simulink model "PSB_FPGAdesign8_model"  (R2021a)
settings: Solver=VariableStepAuto  StartTime=0.0  StopTime=3000  RelTol=1e-3
values from neighbouring files (symbols this model uses):
  n_channel = 1024    [PSB3_0_script.m]    (also in PSB_FPGAdesign8_script.m)
  parallel_factor = 4    [PSB3_0_script.m]    (also in PSB_FPGAdesign8_script.m)
libraries: xbsIndex_r4 x1089, xrbsSSR_Library x150, dspsrcs4 x48
(part 6 of 7)

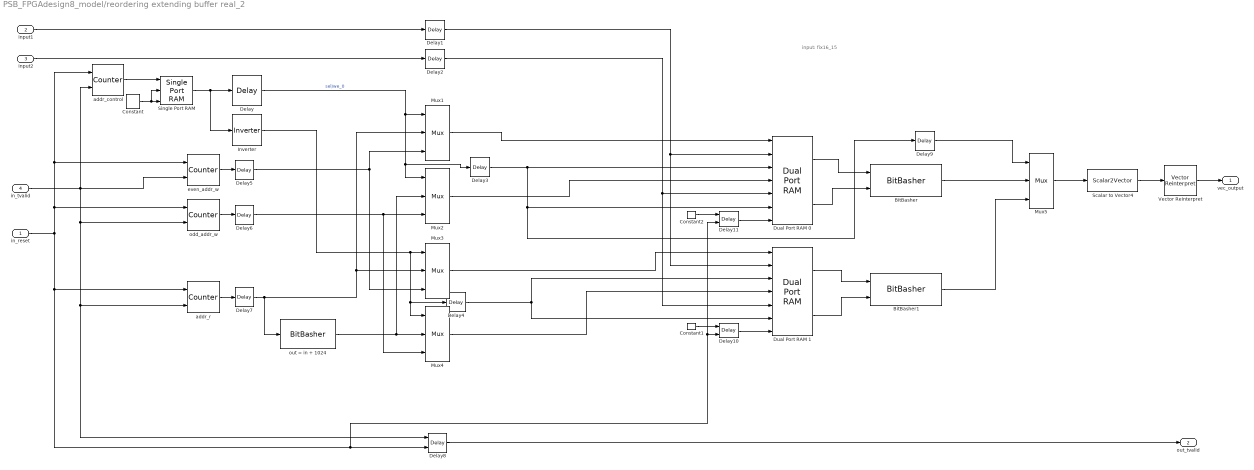
== system PSB_FPGAdesign8_model/reordering extending buffer real_2 ==
  note: input: fix16_15
  in_reset : Inport
  input1 : Inport  Port=2
  input2 : Inport  Port=3
  in_tvalid : Inport  Port=4
  BitBasher : xbsIndex_r4/BitBasher  bitexpr=out = {8{b,a}}  display_expr=on  sr_1=out  arith_type1=Unsigned  bin_pt1=0  sr_2=2  arith_type2=Unsigned  bin_pt2=0  sr_3=3  arith_type3=Unsigned  bin_pt3=0  sr_4=4  arith_type4=Unsigned  bin_pt4=0  dbl_ovrd=off  block_type=bitbasher
  BitBasher1 : xbsIndex_r4/BitBasher  bitexpr=out = {8{b,a}}  display_expr=on  sr_1=out  arith_type1=Unsigned  bin_pt1=0  sr_2=2  arith_type2=Unsigned  bin_pt2=0  sr_3=3  arith_type3=Unsigned  bin_pt3=0  sr_4=4  arith_type4=Unsigned  bin_pt4=0  dbl_ovrd=off  block_type=bitbasher
  Constant : xbsIndex_r4/Constant  const=0  gui_display_data_type=Boolean  arith_type=Boolean  n_bits=16  bin_pt=14  preci_type=Single  exp_width=8  frac_width=24  explicit_period=on  period=1  equ=P=C  opselect=C  inp2=PCIN>>17  opr=+  inp1=P  carry=CIN  dbl_ovrd=off  block_type=constant
  Constant1 : xbsIndex_r4/Constant  const=1  gui_display_data_type=Boolean  arith_type=Boolean  n_bits=16  bin_pt=14  preci_type=Single  exp_width=8  frac_width=24  explicit_period=on  period=1  equ=P=C  opselect=C  inp2=PCIN>>17  opr=+  inp1=P  carry=CIN  dbl_ovrd=off  block_type=constant
  Constant2 : xbsIndex_r4/Constant  const=1  gui_display_data_type=Boolean  arith_type=Boolean  n_bits=16  bin_pt=14  preci_type=Single  exp_width=8  frac_width=24  explicit_period=on  period=1  equ=P=C  opselect=C  inp2=PCIN>>17  opr=+  inp1=P  carry=CIN  dbl_ovrd=off  block_type=constant
  Delay{,3..4,9} (4 alike) : xbsIndex_r4/Delay  rst=off  infoeditControl=Selection of Reset will increase slice count due to use of real FFs and instead of SRLs  en=off  latency=1  reg_retiming=off  dbl_ovrd=off  block_type=delay
  Delay1 : xbsIndex_r4/Delay  rst=off  infoeditControl=Selection of Reset will increase slice count due to use of real FFs and instead of SRLs  en=off  latency=3  reg_retiming=off  dbl_ovrd=off  block_type=delay
  Delay10 : xbsIndex_r4/Delay  rst=on  infoeditControl=Selection of Reset will increase slice count due to use of real FFs and instead of SRLs  en=off  latency=1000  reg_retiming=off  dbl_ovrd=off  block_type=delay
  Delay11 : xbsIndex_r4/Delay  rst=on  infoeditControl=Selection of Reset will increase slice count due to use of real FFs and instead of SRLs  en=off  latency=1000  reg_retiming=off  dbl_ovrd=off  block_type=delay
  Delay2 : xbsIndex_r4/Delay  rst=off  infoeditControl=Selection of Reset will increase slice count due to use of real FFs and instead of SRLs  en=off  latency=3  reg_retiming=off  dbl_ovrd=off  block_type=delay
  Delay5 : xbsIndex_r4/Delay  rst=off  infoeditControl=Selection of Reset will increase slice count due to use of real FFs and instead of SRLs  en=off  latency=2  reg_retiming=off  dbl_ovrd=off  block_type=delay
  Delay6 : xbsIndex_r4/Delay  rst=off  infoeditControl=Selection of Reset will increase slice count due to use of real FFs and instead of SRLs  en=off  latency=2  reg_retiming=off  dbl_ovrd=off  block_type=delay
  Delay7 : xbsIndex_r4/Delay  rst=off  infoeditControl=Selection of Reset will increase slice count due to use of real FFs and instead of SRLs  en=off  latency=2  reg_retiming=off  dbl_ovrd=off  block_type=delay
  Delay8 : xbsIndex_r4/Delay  rst=on  infoeditControl=Selection of Reset will increase slice count due to use of real FFs and instead of SRLs  en=off  latency=4+1024/parallel_factor+1 - 2  reg_retiming=off  dbl_ovrd=off  block_type=delay
  Dual Port RAM 0 : xbsIndex_r4/Dual Port RAM  depth=2048/parallel_factor  initVector=1  distributed_mem=Block RAM  init_a=0  init_b=0  rst_a=off  rst_b=off  en_a=off  en_b=on  latency=1  write_mode_A=Read Before Write  write_mode_B=Read Before Write  optimize=Area  dbl_ovrd=off  simulation_type=fast_sim  block_type=dpram
  Dual Port RAM 1 : xbsIndex_r4/Dual Port RAM  depth=2048/parallel_factor  initVector=1  distributed_mem=Block RAM  init_a=0  init_b=0  rst_a=off  rst_b=off  en_a=off  en_b=on  latency=1  write_mode_A=Read Before Write  write_mode_B=Read Before Write  optimize=Area  dbl_ovrd=off  simulation_type=fast_sim  block_type=dpram
  Inverter : xbsIndex_r4/Inverter  en=off  latency=1  dbl_ovrd=off  block_type=inv
  Mux{1..4} (4 alike) : xbsIndex_r4/Mux  inputs=2  en=off  latency=1  precision=Full  arith_type=Unsigned  n_bits=16  bin_pt=14  quantization=Truncate  overflow=Wrap  dbl_ovrd=off  block_type=mux
  Mux5 : xbsIndex_r4/Mux  inputs=2  en=off  latency=1  precision=User Defined  arith_type=Unsigned  n_bits=256  bin_pt=0  quantization=Truncate  overflow=Flag as error  dbl_ovrd=off  block_type=mux
  Scalar to Vector4 : xrbsSSR_Library/Scalar2Vector  Width=16  sg_ssr=16  sg_ssr_prev=16  sg_ssr_name=vect_Scalar2Vector  block_type=scalar2vector_ssr
      settings: SourceProductName=Xilinx SSR Blockset
  Single Port RAM : xbsIndex_r4/Single Port RAM  depth=2048/parallel_factor  initVector=[ones(1,1024/parallel_factor), zeros(1,1024/parallel_factor)]  distributed_mem=Block RAM  write_mode=Read Before Write  rst=off  init_reg=0  en=off  optimize_latency=off  latency=1  optimize=Area  dbl_ovrd=off  simulation_type=fast_sim  block_type=spram
  Vector Reinterpret : xrbsSSR_Library/Vector Reinterpret  sg_ssr=16  sg_ssr_prev=16  force_arith_type=on  arith_type="Signed  (2's comp)"  force_bin_pt=on  bin_pt=15  block_type=reinterpret_ssr
      settings: SourceProductName=Xilinx SSR Blockset  infoedit="The Vector Reinterpret block Changes vector input signal type without altering the binary representation. You can change the signal between signed and unsigned, and relocate the binary point.<br><br>Hardware notes: In hardware this block costs nothing.<br><br>Example:  Suppose the input is 6 bits wide, signed, with 2 fractional bits, and the output is forced to unsigned with 0 fractional bits.  Then an input of -2.0 (1110.00 in binary 2's complement) becomes an output of 56 (111000 in binary)."
  addr_control : xbsIndex_r4/Counter  cnt_type=Free Running  cnt_to=Inf  operation=Up  start_count=0  cnt_by_val=1  arith_type=Unsigned  n_bits=11-2  bin_pt=0  load_pin=off  rst=on  en=on  explicit_period=on  period=1  use_behavioral_HDL=off  implementation=Fabric  dbl_ovrd=off  block_type=counter
  addr_r : xbsIndex_r4/Counter  cnt_type=Free Running  cnt_to=Inf  operation=Up  start_count=0  cnt_by_val=1  arith_type=Unsigned  n_bits=10-2  bin_pt=0  load_pin=off  rst=on  en=on  explicit_period=on  period=1  use_behavioral_HDL=off  implementation=Fabric  dbl_ovrd=off  block_type=counter
  even_addr_w : xbsIndex_r4/Counter  cnt_type=Free Running  cnt_to=Inf  operation=Up  start_count=0  cnt_by_val=2  arith_type=Unsigned  n_bits=11-2  bin_pt=0  load_pin=off  rst=on  en=on  explicit_period=on  period=1  use_behavioral_HDL=off  implementation=Fabric  dbl_ovrd=off  block_type=counter
  odd_addr_w : xbsIndex_r4/Counter  cnt_type=Free Running  cnt_to=Inf  operation=Up  start_count=1  cnt_by_val=2  arith_type=Unsigned  n_bits=11-2  bin_pt=0  load_pin=off  rst=on  en=on  explicit_period=on  period=1  use_behavioral_HDL=off  implementation=Fabric  dbl_ovrd=off  block_type=counter
  out = in + 1024 : xbsIndex_r4/BitBasher  bitexpr=out={1'b1, in}  display_expr=on  sr_1=out  arith_type1=Unsigned  bin_pt1=0  sr_2=2  arith_type2=Unsigned  bin_pt2=0  sr_3=3  arith_type3=Unsigned  bin_pt3=0  sr_4=4  arith_type4=Unsigned  bin_pt4=0  dbl_ovrd=off  block_type=bitbasher
  vec_output : Outport
  out_tvalid : Outport  Port=2
  wires:
  Delay6/1 -> Mux4/3, Mux2/3
  Dual Port RAM 0/1 -> BitBasher/1
  Delay1/1 -> Dual Port RAM 1/2, Dual Port RAM 0/2
  Mux2/1 -> Dual Port RAM 0/4
  in_tvalid/1 -> addr_r/2, Delay8/1, odd_addr_w/2, even_addr_w/2, addr_control/2
  Mux4/1 -> Dual Port RAM 1/4
  odd_addr_w/1 -> Delay6/1
  Delay9/1 -> Mux5/1
  Delay8/1 -> out_tvalid/1
  Delay/1 -> Delay3/1, Mux2/1, Mux1/1  "sel/we_0"
  even_addr_w/1 -> Delay5/1
  Mux5/1 -> Scalar to Vector4/1
  Mux1/1 -> Dual Port RAM 0/1
  Delay7/1 -> Mux1/2, Mux3/2, out = in + 1024/1
  addr_r/1 -> Delay7/1
  Dual Port RAM 1/1 -> BitBasher1/1
  Mux3/1 -> Dual Port RAM 1/1
  Single Port RAM/1 -> Inverter/1, Delay/1
  Delay3/1 -> Dual Port RAM 0/3, Dual Port RAM 0/6, Delay9/1
  Inverter/1 -> Delay4/1, Mux4/1, Mux3/1
  Constant/1 -> Single Port RAM/2, Single Port RAM/3
  out = in + 1024/1 -> Mux2/2, Mux4/2
  Delay2/1 -> Dual Port RAM 1/5, Dual Port RAM 0/5
  addr_control/1 -> Single Port RAM/1
  Delay5/1 -> Mux3/3, Mux1/3
  BitBasher/1 -> Mux5/2
  Delay4/1 -> Dual Port RAM 1/6, Dual Port RAM 1/3
  BitBasher1/1 -> Mux5/3
  Scalar to Vector4/1 -> Vector Reinterpret/1
  input1/1 -> Delay1/1
  input2/1 -> Delay2/1
  Constant2/1 -> Delay11/1
  Delay11/1 -> Dual Port RAM 0/7
  Constant1/1 -> Delay10/1
  Delay10/1 -> Dual Port RAM 1/7
  Dual Port RAM 0/2 -> BitBasher/2
  Dual Port RAM 1/2 -> BitBasher1/2
  Vector Reinterpret/1 -> vec_output/1
  in_reset/1 -> Delay11/2, Delay10/2, Delay8/2, addr_r/1, odd_addr_w/1, even_addr_w/1, addr_control/1

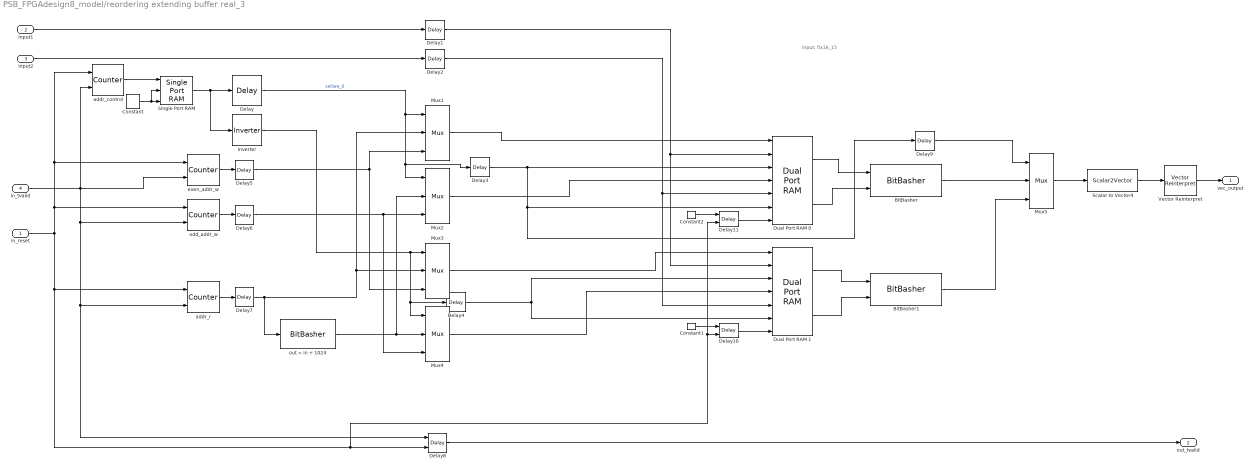
== system PSB_FPGAdesign8_model/reordering extending buffer real_3 ==
  note: input: fix16_15
  in_reset : Inport
  input1 : Inport  Port=2
  input2 : Inport  Port=3
  in_tvalid : Inport  Port=4
  BitBasher : xbsIndex_r4/BitBasher  bitexpr=out = {8{b,a}}  display_expr=on  sr_1=out  arith_type1=Unsigned  bin_pt1=0  sr_2=2  arith_type2=Unsigned  bin_pt2=0  sr_3=3  arith_type3=Unsigned  bin_pt3=0  sr_4=4  arith_type4=Unsigned  bin_pt4=0  dbl_ovrd=off  block_type=bitbasher
  BitBasher1 : xbsIndex_r4/BitBasher  bitexpr=out = {8{b,a}}  display_expr=on  sr_1=out  arith_type1=Unsigned  bin_pt1=0  sr_2=2  arith_type2=Unsigned  bin_pt2=0  sr_3=3  arith_type3=Unsigned  bin_pt3=0  sr_4=4  arith_type4=Unsigned  bin_pt4=0  dbl_ovrd=off  block_type=bitbasher
  Constant : xbsIndex_r4/Constant  const=0  gui_display_data_type=Boolean  arith_type=Boolean  n_bits=16  bin_pt=14  preci_type=Single  exp_width=8  frac_width=24  explicit_period=on  period=1  equ=P=C  opselect=C  inp2=PCIN>>17  opr=+  inp1=P  carry=CIN  dbl_ovrd=off  block_type=constant
  Constant1 : xbsIndex_r4/Constant  const=1  gui_display_data_type=Boolean  arith_type=Boolean  n_bits=16  bin_pt=14  preci_type=Single  exp_width=8  frac_width=24  explicit_period=on  period=1  equ=P=C  opselect=C  inp2=PCIN>>17  opr=+  inp1=P  carry=CIN  dbl_ovrd=off  block_type=constant
  Constant2 : xbsIndex_r4/Constant  const=1  gui_display_data_type=Boolean  arith_type=Boolean  n_bits=16  bin_pt=14  preci_type=Single  exp_width=8  frac_width=24  explicit_period=on  period=1  equ=P=C  opselect=C  inp2=PCIN>>17  opr=+  inp1=P  carry=CIN  dbl_ovrd=off  block_type=constant
  Delay{,3..4,9} (4 alike) : xbsIndex_r4/Delay  rst=off  infoeditControl=Selection of Reset will increase slice count due to use of real FFs and instead of SRLs  en=off  latency=1  reg_retiming=off  dbl_ovrd=off  block_type=delay
  Delay1 : xbsIndex_r4/Delay  rst=off  infoeditControl=Selection of Reset will increase slice count due to use of real FFs and instead of SRLs  en=off  latency=3  reg_retiming=off  dbl_ovrd=off  block_type=delay
  Delay10 : xbsIndex_r4/Delay  rst=on  infoeditControl=Selection of Reset will increase slice count due to use of real FFs and instead of SRLs  en=off  latency=1000  reg_retiming=off  dbl_ovrd=off  block_type=delay
  Delay11 : xbsIndex_r4/Delay  rst=on  infoeditControl=Selection of Reset will increase slice count due to use of real FFs and instead of SRLs  en=off  latency=1000  reg_retiming=off  dbl_ovrd=off  block_type=delay
  Delay2 : xbsIndex_r4/Delay  rst=off  infoeditControl=Selection of Reset will increase slice count due to use of real FFs and instead of SRLs  en=off  latency=3  reg_retiming=off  dbl_ovrd=off  block_type=delay
  Delay5 : xbsIndex_r4/Delay  rst=off  infoeditControl=Selection of Reset will increase slice count due to use of real FFs and instead of SRLs  en=off  latency=2  reg_retiming=off  dbl_ovrd=off  block_type=delay
  Delay6 : xbsIndex_r4/Delay  rst=off  infoeditControl=Selection of Reset will increase slice count due to use of real FFs and instead of SRLs  en=off  latency=2  reg_retiming=off  dbl_ovrd=off  block_type=delay
  Delay7 : xbsIndex_r4/Delay  rst=off  infoeditControl=Selection of Reset will increase slice count due to use of real FFs and instead of SRLs  en=off  latency=2  reg_retiming=off  dbl_ovrd=off  block_type=delay
  Delay8 : xbsIndex_r4/Delay  rst=on  infoeditControl=Selection of Reset will increase slice count due to use of real FFs and instead of SRLs  en=off  latency=4+1024/parallel_factor+1 - 2  reg_retiming=off  dbl_ovrd=off  block_type=delay
  Dual Port RAM 0 : xbsIndex_r4/Dual Port RAM  depth=2048/parallel_factor  initVector=1  distributed_mem=Block RAM  init_a=0  init_b=0  rst_a=off  rst_b=off  en_a=off  en_b=on  latency=1  write_mode_A=Read Before Write  write_mode_B=Read Before Write  optimize=Area  dbl_ovrd=off  simulation_type=fast_sim  block_type=dpram
  Dual Port RAM 1 : xbsIndex_r4/Dual Port RAM  depth=2048/parallel_factor  initVector=1  distributed_mem=Block RAM  init_a=0  init_b=0  rst_a=off  rst_b=off  en_a=off  en_b=on  latency=1  write_mode_A=Read Before Write  write_mode_B=Read Before Write  optimize=Area  dbl_ovrd=off  simulation_type=fast_sim  block_type=dpram
  Inverter : xbsIndex_r4/Inverter  en=off  latency=1  dbl_ovrd=off  block_type=inv
  Mux{1..4} (4 alike) : xbsIndex_r4/Mux  inputs=2  en=off  latency=1  precision=Full  arith_type=Unsigned  n_bits=16  bin_pt=14  quantization=Truncate  overflow=Wrap  dbl_ovrd=off  block_type=mux
  Mux5 : xbsIndex_r4/Mux  inputs=2  en=off  latency=1  precision=User Defined  arith_type=Unsigned  n_bits=256  bin_pt=0  quantization=Truncate  overflow=Flag as error  dbl_ovrd=off  block_type=mux
  Scalar to Vector4 : xrbsSSR_Library/Scalar2Vector  Width=16  sg_ssr=16  sg_ssr_prev=16  sg_ssr_name=vect_Scalar2Vector  block_type=scalar2vector_ssr
      settings: SourceProductName=Xilinx SSR Blockset
  Single Port RAM : xbsIndex_r4/Single Port RAM  depth=2048/parallel_factor  initVector=[ones(1,1024/parallel_factor), zeros(1,1024/parallel_factor)]  distributed_mem=Block RAM  write_mode=Read Before Write  rst=off  init_reg=0  en=off  optimize_latency=off  latency=1  optimize=Area  dbl_ovrd=off  simulation_type=fast_sim  block_type=spram
  Vector Reinterpret : xrbsSSR_Library/Vector Reinterpret  sg_ssr=16  sg_ssr_prev=16  force_arith_type=on  arith_type="Signed  (2's comp)"  force_bin_pt=on  bin_pt=15  block_type=reinterpret_ssr
      settings: SourceProductName=Xilinx SSR Blockset  infoedit="The Vector Reinterpret block Changes vector input signal type without altering the binary representation. You can change the signal between signed and unsigned, and relocate the binary point.<br><br>Hardware notes: In hardware this block costs nothing.<br><br>Example:  Suppose the input is 6 bits wide, signed, with 2 fractional bits, and the output is forced to unsigned with 0 fractional bits.  Then an input of -2.0 (1110.00 in binary 2's complement) becomes an output of 56 (111000 in binary)."
  addr_control : xbsIndex_r4/Counter  cnt_type=Free Running  cnt_to=Inf  operation=Up  start_count=0  cnt_by_val=1  arith_type=Unsigned  n_bits=11-2  bin_pt=0  load_pin=off  rst=on  en=on  explicit_period=on  period=1  use_behavioral_HDL=off  implementation=Fabric  dbl_ovrd=off  block_type=counter
  addr_r : xbsIndex_r4/Counter  cnt_type=Free Running  cnt_to=Inf  operation=Up  start_count=0  cnt_by_val=1  arith_type=Unsigned  n_bits=10-2  bin_pt=0  load_pin=off  rst=on  en=on  explicit_period=on  period=1  use_behavioral_HDL=off  implementation=Fabric  dbl_ovrd=off  block_type=counter
  even_addr_w : xbsIndex_r4/Counter  cnt_type=Free Running  cnt_to=Inf  operation=Up  start_count=0  cnt_by_val=2  arith_type=Unsigned  n_bits=11-2  bin_pt=0  load_pin=off  rst=on  en=on  explicit_period=on  period=1  use_behavioral_HDL=off  implementation=Fabric  dbl_ovrd=off  block_type=counter
  odd_addr_w : xbsIndex_r4/Counter  cnt_type=Free Running  cnt_to=Inf  operation=Up  start_count=1  cnt_by_val=2  arith_type=Unsigned  n_bits=11-2  bin_pt=0  load_pin=off  rst=on  en=on  explicit_period=on  period=1  use_behavioral_HDL=off  implementation=Fabric  dbl_ovrd=off  block_type=counter
  out = in + 1024 : xbsIndex_r4/BitBasher  bitexpr=out={1'b1, in}  display_expr=on  sr_1=out  arith_type1=Unsigned  bin_pt1=0  sr_2=2  arith_type2=Unsigned  bin_pt2=0  sr_3=3  arith_type3=Unsigned  bin_pt3=0  sr_4=4  arith_type4=Unsigned  bin_pt4=0  dbl_ovrd=off  block_type=bitbasher
  vec_output : Outport
  out_tvalid : Outport  Port=2
  wires:
  Delay6/1 -> Mux4/3, Mux2/3
  Dual Port RAM 0/1 -> BitBasher/1
  Delay1/1 -> Dual Port RAM 1/2, Dual Port RAM 0/2
  Mux2/1 -> Dual Port RAM 0/4
  in_tvalid/1 -> addr_r/2, Delay8/1, odd_addr_w/2, even_addr_w/2, addr_control/2
  Mux4/1 -> Dual Port RAM 1/4
  odd_addr_w/1 -> Delay6/1
  Delay9/1 -> Mux5/1
  Delay8/1 -> out_tvalid/1
  Delay/1 -> Delay3/1, Mux2/1, Mux1/1  "sel/we_0"
  even_addr_w/1 -> Delay5/1
  Mux5/1 -> Scalar to Vector4/1
  Mux1/1 -> Dual Port RAM 0/1
  Delay7/1 -> Mux1/2, Mux3/2, out = in + 1024/1
  addr_r/1 -> Delay7/1
  Dual Port RAM 1/1 -> BitBasher1/1
  Mux3/1 -> Dual Port RAM 1/1
  Single Port RAM/1 -> Inverter/1, Delay/1
  Delay3/1 -> Dual Port RAM 0/3, Dual Port RAM 0/6, Delay9/1
  Inverter/1 -> Delay4/1, Mux4/1, Mux3/1
  Constant/1 -> Single Port RAM/2, Single Port RAM/3
  out = in + 1024/1 -> Mux2/2, Mux4/2
  Delay2/1 -> Dual Port RAM 1/5, Dual Port RAM 0/5
  addr_control/1 -> Single Port RAM/1
  Delay5/1 -> Mux3/3, Mux1/3
  BitBasher/1 -> Mux5/2
  Delay4/1 -> Dual Port RAM 1/6, Dual Port RAM 1/3
  BitBasher1/1 -> Mux5/3
  Scalar to Vector4/1 -> Vector Reinterpret/1
  input1/1 -> Delay1/1
  input2/1 -> Delay2/1
  Constant2/1 -> Delay11/1
  Delay11/1 -> Dual Port RAM 0/7
  Constant1/1 -> Delay10/1
  Delay10/1 -> Dual Port RAM 1/7
  Dual Port RAM 0/2 -> BitBasher/2
  Dual Port RAM 1/2 -> BitBasher1/2
  Vector Reinterpret/1 -> vec_output/1
  in_reset/1 -> Delay11/2, Delay10/2, Delay8/2, addr_r/1, odd_addr_w/1, even_addr_w/1, addr_control/1

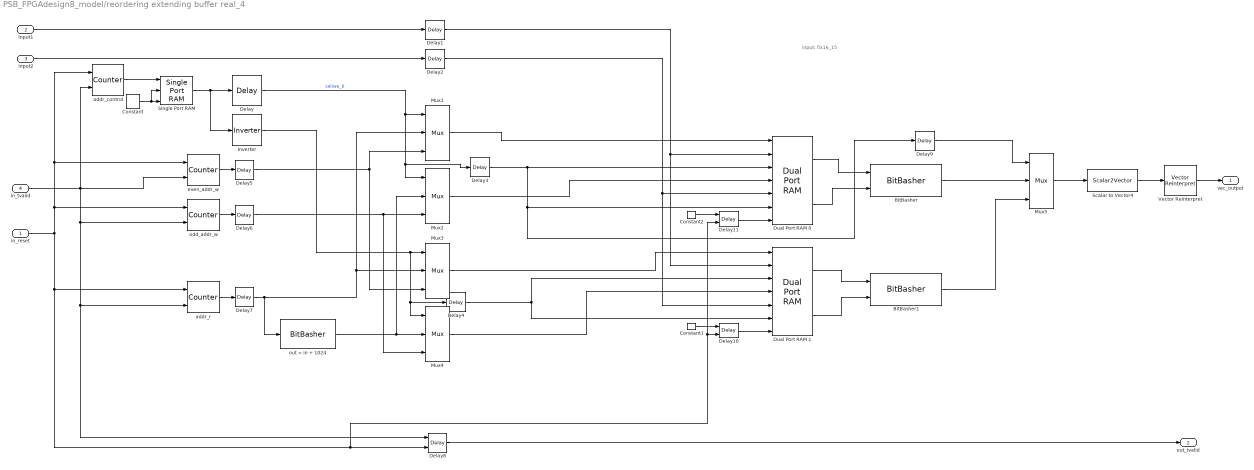
== system PSB_FPGAdesign8_model/reordering extending buffer real_4 ==
  note: input: fix16_15
  in_reset : Inport
  input1 : Inport  Port=2
  input2 : Inport  Port=3
  in_tvalid : Inport  Port=4
  BitBasher : xbsIndex_r4/BitBasher  bitexpr=out = {8{b,a}}  display_expr=on  sr_1=out  arith_type1=Unsigned  bin_pt1=0  sr_2=2  arith_type2=Unsigned  bin_pt2=0  sr_3=3  arith_type3=Unsigned  bin_pt3=0  sr_4=4  arith_type4=Unsigned  bin_pt4=0  dbl_ovrd=off  block_type=bitbasher
  BitBasher1 : xbsIndex_r4/BitBasher  bitexpr=out = {8{b,a}}  display_expr=on  sr_1=out  arith_type1=Unsigned  bin_pt1=0  sr_2=2  arith_type2=Unsigned  bin_pt2=0  sr_3=3  arith_type3=Unsigned  bin_pt3=0  sr_4=4  arith_type4=Unsigned  bin_pt4=0  dbl_ovrd=off  block_type=bitbasher
  Constant : xbsIndex_r4/Constant  const=0  gui_display_data_type=Boolean  arith_type=Boolean  n_bits=16  bin_pt=14  preci_type=Single  exp_width=8  frac_width=24  explicit_period=on  period=1  equ=P=C  opselect=C  inp2=PCIN>>17  opr=+  inp1=P  carry=CIN  dbl_ovrd=off  block_type=constant
  Constant1 : xbsIndex_r4/Constant  const=1  gui_display_data_type=Boolean  arith_type=Boolean  n_bits=16  bin_pt=14  preci_type=Single  exp_width=8  frac_width=24  explicit_period=on  period=1  equ=P=C  opselect=C  inp2=PCIN>>17  opr=+  inp1=P  carry=CIN  dbl_ovrd=off  block_type=constant
  Constant2 : xbsIndex_r4/Constant  const=1  gui_display_data_type=Boolean  arith_type=Boolean  n_bits=16  bin_pt=14  preci_type=Single  exp_width=8  frac_width=24  explicit_period=on  period=1  equ=P=C  opselect=C  inp2=PCIN>>17  opr=+  inp1=P  carry=CIN  dbl_ovrd=off  block_type=constant
  Delay{,3..4,9} (4 alike) : xbsIndex_r4/Delay  rst=off  infoeditControl=Selection of Reset will increase slice count due to use of real FFs and instead of SRLs  en=off  latency=1  reg_retiming=off  dbl_ovrd=off  block_type=delay
  Delay1 : xbsIndex_r4/Delay  rst=off  infoeditControl=Selection of Reset will increase slice count due to use of real FFs and instead of SRLs  en=off  latency=3  reg_retiming=off  dbl_ovrd=off  block_type=delay
  Delay10 : xbsIndex_r4/Delay  rst=on  infoeditControl=Selection of Reset will increase slice count due to use of real FFs and instead of SRLs  en=off  latency=1000  reg_retiming=off  dbl_ovrd=off  block_type=delay
  Delay11 : xbsIndex_r4/Delay  rst=on  infoeditControl=Selection of Reset will increase slice count due to use of real FFs and instead of SRLs  en=off  latency=1000  reg_retiming=off  dbl_ovrd=off  block_type=delay
  Delay2 : xbsIndex_r4/Delay  rst=off  infoeditControl=Selection of Reset will increase slice count due to use of real FFs and instead of SRLs  en=off  latency=3  reg_retiming=off  dbl_ovrd=off  block_type=delay
  Delay5 : xbsIndex_r4/Delay  rst=off  infoeditControl=Selection of Reset will increase slice count due to use of real FFs and instead of SRLs  en=off  latency=2  reg_retiming=off  dbl_ovrd=off  block_type=delay
  Delay6 : xbsIndex_r4/Delay  rst=off  infoeditControl=Selection of Reset will increase slice count due to use of real FFs and instead of SRLs  en=off  latency=2  reg_retiming=off  dbl_ovrd=off  block_type=delay
  Delay7 : xbsIndex_r4/Delay  rst=off  infoeditControl=Selection of Reset will increase slice count due to use of real FFs and instead of SRLs  en=off  latency=2  reg_retiming=off  dbl_ovrd=off  block_type=delay
  Delay8 : xbsIndex_r4/Delay  rst=on  infoeditControl=Selection of Reset will increase slice count due to use of real FFs and instead of SRLs  en=off  latency=4+1024/parallel_factor+1 - 2  reg_retiming=off  dbl_ovrd=off  block_type=delay
  Dual Port RAM 0 : xbsIndex_r4/Dual Port RAM  depth=2048/parallel_factor  initVector=1  distributed_mem=Block RAM  init_a=0  init_b=0  rst_a=off  rst_b=off  en_a=off  en_b=on  latency=1  write_mode_A=Read Before Write  write_mode_B=Read Before Write  optimize=Area  dbl_ovrd=off  simulation_type=fast_sim  block_type=dpram
  Dual Port RAM 1 : xbsIndex_r4/Dual Port RAM  depth=2048/parallel_factor  initVector=1  distributed_mem=Block RAM  init_a=0  init_b=0  rst_a=off  rst_b=off  en_a=off  en_b=on  latency=1  write_mode_A=Read Before Write  write_mode_B=Read Before Write  optimize=Area  dbl_ovrd=off  simulation_type=fast_sim  block_type=dpram
  Inverter : xbsIndex_r4/Inverter  en=off  latency=1  dbl_ovrd=off  block_type=inv
  Mux{1..4} (4 alike) : xbsIndex_r4/Mux  inputs=2  en=off  latency=1  precision=Full  arith_type=Unsigned  n_bits=16  bin_pt=14  quantization=Truncate  overflow=Wrap  dbl_ovrd=off  block_type=mux
  Mux5 : xbsIndex_r4/Mux  inputs=2  en=off  latency=1  precision=User Defined  arith_type=Unsigned  n_bits=256  bin_pt=0  quantization=Truncate  overflow=Flag as error  dbl_ovrd=off  block_type=mux
  Scalar to Vector4 : xrbsSSR_Library/Scalar2Vector  Width=16  sg_ssr=16  sg_ssr_prev=16  sg_ssr_name=vect_Scalar2Vector  block_type=scalar2vector_ssr
      settings: SourceProductName=Xilinx SSR Blockset
  Single Port RAM : xbsIndex_r4/Single Port RAM  depth=2048/parallel_factor  initVector=[ones(1,1024/parallel_factor), zeros(1,1024/parallel_factor)]  distributed_mem=Block RAM  write_mode=Read Before Write  rst=off  init_reg=0  en=off  optimize_latency=off  latency=1  optimize=Area  dbl_ovrd=off  simulation_type=fast_sim  block_type=spram
  Vector Reinterpret : xrbsSSR_Library/Vector Reinterpret  sg_ssr=16  sg_ssr_prev=16  force_arith_type=on  arith_type="Signed  (2's comp)"  force_bin_pt=on  bin_pt=15  block_type=reinterpret_ssr
      settings: SourceProductName=Xilinx SSR Blockset  infoedit="The Vector Reinterpret block Changes vector input signal type without altering the binary representation. You can change the signal between signed and unsigned, and relocate the binary point.<br><br>Hardware notes: In hardware this block costs nothing.<br><br>Example:  Suppose the input is 6 bits wide, signed, with 2 fractional bits, and the output is forced to unsigned with 0 fractional bits.  Then an input of -2.0 (1110.00 in binary 2's complement) becomes an output of 56 (111000 in binary)."
  addr_control : xbsIndex_r4/Counter  cnt_type=Free Running  cnt_to=Inf  operation=Up  start_count=0  cnt_by_val=1  arith_type=Unsigned  n_bits=11-2  bin_pt=0  load_pin=off  rst=on  en=on  explicit_period=on  period=1  use_behavioral_HDL=off  implementation=Fabric  dbl_ovrd=off  block_type=counter
  addr_r : xbsIndex_r4/Counter  cnt_type=Free Running  cnt_to=Inf  operation=Up  start_count=0  cnt_by_val=1  arith_type=Unsigned  n_bits=10-2  bin_pt=0  load_pin=off  rst=on  en=on  explicit_period=on  period=1  use_behavioral_HDL=off  implementation=Fabric  dbl_ovrd=off  block_type=counter
  even_addr_w : xbsIndex_r4/Counter  cnt_type=Free Running  cnt_to=Inf  operation=Up  start_count=0  cnt_by_val=2  arith_type=Unsigned  n_bits=11-2  bin_pt=0  load_pin=off  rst=on  en=on  explicit_period=on  period=1  use_behavioral_HDL=off  implementation=Fabric  dbl_ovrd=off  block_type=counter
  odd_addr_w : xbsIndex_r4/Counter  cnt_type=Free Running  cnt_to=Inf  operation=Up  start_count=1  cnt_by_val=2  arith_type=Unsigned  n_bits=11-2  bin_pt=0  load_pin=off  rst=on  en=on  explicit_period=on  period=1  use_behavioral_HDL=off  implementation=Fabric  dbl_ovrd=off  block_type=counter
  out = in + 1024 : xbsIndex_r4/BitBasher  bitexpr=out={1'b1, in}  display_expr=on  sr_1=out  arith_type1=Unsigned  bin_pt1=0  sr_2=2  arith_type2=Unsigned  bin_pt2=0  sr_3=3  arith_type3=Unsigned  bin_pt3=0  sr_4=4  arith_type4=Unsigned  bin_pt4=0  dbl_ovrd=off  block_type=bitbasher
  vec_output : Outport
  out_tvalid : Outport  Port=2
  wires:
  Delay6/1 -> Mux4/3, Mux2/3
  Dual Port RAM 0/1 -> BitBasher/1
  Delay1/1 -> Dual Port RAM 1/2, Dual Port RAM 0/2
  Mux2/1 -> Dual Port RAM 0/4
  in_tvalid/1 -> addr_r/2, Delay8/1, odd_addr_w/2, even_addr_w/2, addr_control/2
  Mux4/1 -> Dual Port RAM 1/4
  odd_addr_w/1 -> Delay6/1
  Delay9/1 -> Mux5/1
  Delay8/1 -> out_tvalid/1
  Delay/1 -> Delay3/1, Mux2/1, Mux1/1  "sel/we_0"
  even_addr_w/1 -> Delay5/1
  Mux5/1 -> Scalar to Vector4/1
  Mux1/1 -> Dual Port RAM 0/1
  Delay7/1 -> Mux1/2, Mux3/2, out = in + 1024/1
  addr_r/1 -> Delay7/1
  Dual Port RAM 1/1 -> BitBasher1/1
  Mux3/1 -> Dual Port RAM 1/1
  Single Port RAM/1 -> Inverter/1, Delay/1
  Delay3/1 -> Dual Port RAM 0/3, Dual Port RAM 0/6, Delay9/1
  Inverter/1 -> Delay4/1, Mux4/1, Mux3/1
  Constant/1 -> Single Port RAM/2, Single Port RAM/3
  out = in + 1024/1 -> Mux2/2, Mux4/2
  Delay2/1 -> Dual Port RAM 1/5, Dual Port RAM 0/5
  addr_control/1 -> Single Port RAM/1
  Delay5/1 -> Mux3/3, Mux1/3
  BitBasher/1 -> Mux5/2
  Delay4/1 -> Dual Port RAM 1/6, Dual Port RAM 1/3
  BitBasher1/1 -> Mux5/3
  Scalar to Vector4/1 -> Vector Reinterpret/1
  input1/1 -> Delay1/1
  input2/1 -> Delay2/1
  Constant2/1 -> Delay11/1
  Delay11/1 -> Dual Port RAM 0/7
  Constant1/1 -> Delay10/1
  Delay10/1 -> Dual Port RAM 1/7
  Dual Port RAM 0/2 -> BitBasher/2
  Dual Port RAM 1/2 -> BitBasher1/2
  Vector Reinterpret/1 -> vec_output/1
  in_reset/1 -> Delay11/2, Delay10/2, Delay8/2, addr_r/1, odd_addr_w/1, even_addr_w/1, addr_control/1

== system PSB_FPGAdesign8_model/vector IFFT ==
  note: For the output precision parameter of this block,
      | the output bitwidth sets the output bit width, affects FFT computation precision/overflow
      | the binary point parameter is used for reinterpret, must be 14 for unscaled value
      | For example, if the output binary point is 15, the output values are effectively right shifted by 1.
  I.RE : Inport
  I.IM : Inport  Port=2
  VI : Inport  Port=3
  SI : Inport  Port=4
  Vector FFT : xrbsSSR_Library/Vector FFT  sg_ssr=8  N=2048  W_high=1  W_low=-17  n_bits=20  bin_pt=14+1  bram_threshold=258  block_type=fft_ssr  sg_ssr_prev=8
      settings: SourceProductName=Xilinx SSR Blockset
  O.RE : Outport
  O.IM : Outport  Port=2
  VO : Outport  Port=3
  SO : Outport  Port=4
  wires:
  Vector FFT/3 -> VO/1
  Vector FFT/4 -> SO/1
  SI/1 -> Vector FFT/4
  VI/1 -> Vector FFT/3
  Vector FFT/2 -> O.RE/1
  Vector FFT/1 -> O.IM/1
  I.RE/1 -> Vector FFT/2
  I.IM/1 -> Vector FFT/1

== system PSB_FPGAdesign8_model/Baseband_even_1/delayCounter2 ==
  note: Counter that is enabled after the first rising edge1, and disabled after the first rising edge2. Need to calibrate the initial value of counter before getting desired delay value.
  edge1 : Inport
  edge2 : Inport  Port=2
  Counter1 : xbsIndex_r4/Counter  cnt_type=Free Running  cnt_to=Inf  operation=Up  start_count=0  cnt_by_val=1  arith_type=Unsigned  n_bits=12  bin_pt=0  load_pin=off  rst=off  en=on  explicit_period=on  period=1  use_behavioral_HDL=off  implementation=DSP48  dbl_ovrd=off  block_type=counter
  Logical : xbsIndex_r4/Logical  logical_function=XOR  inputs=2  en=off  latency=1  precision=User Defined  arith_type=Boolean  n_bits=1  bin_pt=0  align_bp=on  dbl_ovrd=off  block_type=logical
  Register1 : xbsIndex_r4/Register  init=0  rst=off  en=on  dbl_ovrd=off  block_type=register
  Register2 : xbsIndex_r4/Register  init=0  rst=off  en=on  dbl_ovrd=off  block_type=register
  const1 : xbsIndex_r4/Constant  const=1  gui_display_data_type=Boolean  arith_type=Boolean  n_bits=18  bin_pt=16  preci_type=Single  exp_width=8  frac_width=24  explicit_period=on  period=1  equ=P=C  opselect=C  inp2=PCIN>>17  opr=+  inp1=P  carry=CIN  dbl_ovrd=off  block_type=constant
  delay : Outport
  wires:
  Counter1/1 -> delay/1
  Register2/1 -> Logical/2
  Logical/1 -> Counter1/1
  const1/1 -> Register1/1, Register2/1
  Register1/1 -> Logical/1
  edge2/1 -> Register2/2
  edge1/1 -> Register1/2

== system PSB_FPGAdesign8_model/Baseband_even_2/delayCounter_even_2 ==
  note: Counter that is enabled after the first rising edge1, and disabled after the first rising edge2. Need to calibrate the initial value of counter before getting desired delay value.
  edge1 : Inport
  edge2 : Inport  Port=2
  Counter1 : xbsIndex_r4/Counter  cnt_type=Free Running  cnt_to=Inf  operation=Up  start_count=0  cnt_by_val=1  arith_type=Unsigned  n_bits=12  bin_pt=0  load_pin=off  rst=off  en=on  explicit_period=on  period=1  use_behavioral_HDL=off  implementation=DSP48  dbl_ovrd=off  block_type=counter
  Logical : xbsIndex_r4/Logical  logical_function=XOR  inputs=2  en=off  latency=1  precision=User Defined  arith_type=Boolean  n_bits=1  bin_pt=0  align_bp=on  dbl_ovrd=off  block_type=logical
  Register1 : xbsIndex_r4/Register  init=0  rst=off  en=on  dbl_ovrd=off  block_type=register
  Register2 : xbsIndex_r4/Register  init=0  rst=off  en=on  dbl_ovrd=off  block_type=register
  const1 : xbsIndex_r4/Constant  const=1  gui_display_data_type=Boolean  arith_type=Boolean  n_bits=18  bin_pt=16  preci_type=Single  exp_width=8  frac_width=24  explicit_period=on  period=1  equ=P=C  opselect=C  inp2=PCIN>>17  opr=+  inp1=P  carry=CIN  dbl_ovrd=off  block_type=constant
  delay : Outport
  wires:
  edge1/1 -> Register1/2
  edge2/1 -> Register2/2
  Register1/1 -> Logical/1
  const1/1 -> Register2/1, Register1/1
  Logical/1 -> Counter1/1
  Register2/1 -> Logical/2
  Counter1/1 -> delay/1

== system PSB_FPGAdesign8_model/Baseband_even_3/delayCounter2 ==
  note: Counter that is enabled after the first rising edge1, and disabled after the first rising edge2. Need to calibrate the initial value of counter before getting desired delay value.
  edge1 : Inport
  edge2 : Inport  Port=2
  Counter1 : xbsIndex_r4/Counter  cnt_type=Free Running  cnt_to=Inf  operation=Up  start_count=0  cnt_by_val=1  arith_type=Unsigned  n_bits=12  bin_pt=0  load_pin=off  rst=off  en=on  explicit_period=on  period=1  use_behavioral_HDL=off  implementation=DSP48  dbl_ovrd=off  block_type=counter
  Logical : xbsIndex_r4/Logical  logical_function=XOR  inputs=2  en=off  latency=1  precision=User Defined  arith_type=Boolean  n_bits=1  bin_pt=0  align_bp=on  dbl_ovrd=off  block_type=logical
  Register1 : xbsIndex_r4/Register  init=0  rst=off  en=on  dbl_ovrd=off  block_type=register
  Register2 : xbsIndex_r4/Register  init=0  rst=off  en=on  dbl_ovrd=off  block_type=register
  const1 : xbsIndex_r4/Constant  const=1  gui_display_data_type=Boolean  arith_type=Boolean  n_bits=18  bin_pt=16  preci_type=Single  exp_width=8  frac_width=24  explicit_period=on  period=1  equ=P=C  opselect=C  inp2=PCIN>>17  opr=+  inp1=P  carry=CIN  dbl_ovrd=off  block_type=constant
  delay : Outport
  wires:
  edge1/1 -> Register1/2
  edge2/1 -> Register2/2
  Register1/1 -> Logical/1
  const1/1 -> Register2/1, Register1/1
  Logical/1 -> Counter1/1
  Register2/1 -> Logical/2
  Counter1/1 -> delay/1

== system PSB_FPGAdesign8_model/Baseband_even_4/delayCounter_even_2 ==
  note: Counter that is enabled after the first rising edge1, and disabled after the first rising edge2. Need to calibrate the initial value of counter before getting desired delay value.
  edge1 : Inport
  edge2 : Inport  Port=2
  Counter1 : xbsIndex_r4/Counter  cnt_type=Free Running  cnt_to=Inf  operation=Up  start_count=0  cnt_by_val=1  arith_type=Unsigned  n_bits=12  bin_pt=0  load_pin=off  rst=off  en=on  explicit_period=on  period=1  use_behavioral_HDL=off  implementation=DSP48  dbl_ovrd=off  block_type=counter
  Logical : xbsIndex_r4/Logical  logical_function=XOR  inputs=2  en=off  latency=1  precision=User Defined  arith_type=Boolean  n_bits=1  bin_pt=0  align_bp=on  dbl_ovrd=off  block_type=logical
  Register1 : xbsIndex_r4/Register  init=0  rst=off  en=on  dbl_ovrd=off  block_type=register
  Register2 : xbsIndex_r4/Register  init=0  rst=off  en=on  dbl_ovrd=off  block_type=register
  const1 : xbsIndex_r4/Constant  const=1  gui_display_data_type=Boolean  arith_type=Boolean  n_bits=18  bin_pt=16  preci_type=Single  exp_width=8  frac_width=24  explicit_period=on  period=1  equ=P=C  opselect=C  inp2=PCIN>>17  opr=+  inp1=P  carry=CIN  dbl_ovrd=off  block_type=constant
  delay : Outport
  wires:
  Counter1/1 -> delay/1
  Register2/1 -> Logical/2
  Logical/1 -> Counter1/1
  const1/1 -> Register1/1, Register2/1
  Register1/1 -> Logical/1
  edge2/1 -> Register2/2
  edge1/1 -> Register1/2

== system PSB_FPGAdesign8_model/Baseband_odd_1/delayCounter1 ==
  note: Counter that is enabled after the first rising edge1, and disabled after the first rising edge2. Need to calibrate the initial value of counter before getting desired delay value.
  edge1 : Inport
  edge2 : Inport  Port=2
  Counter1 : xbsIndex_r4/Counter  cnt_type=Free Running  cnt_to=Inf  operation=Up  start_count=0  cnt_by_val=1  arith_type=Unsigned  n_bits=12  bin_pt=0  load_pin=off  rst=off  en=on  explicit_period=on  period=1  use_behavioral_HDL=off  implementation=DSP48  dbl_ovrd=off  block_type=counter
  Logical : xbsIndex_r4/Logical  logical_function=XOR  inputs=2  en=off  latency=1  precision=User Defined  arith_type=Boolean  n_bits=1  bin_pt=0  align_bp=on  dbl_ovrd=off  block_type=logical
  Register1 : xbsIndex_r4/Register  init=0  rst=off  en=on  dbl_ovrd=off  block_type=register
  Register2 : xbsIndex_r4/Register  init=0  rst=off  en=on  dbl_ovrd=off  block_type=register
  const1 : xbsIndex_r4/Constant  const=1  gui_display_data_type=Boolean  arith_type=Boolean  n_bits=18  bin_pt=16  preci_type=Single  exp_width=8  frac_width=24  explicit_period=on  period=1  equ=P=C  opselect=C  inp2=PCIN>>17  opr=+  inp1=P  carry=CIN  dbl_ovrd=off  block_type=constant
  delay : Outport
  wires:
  Counter1/1 -> delay/1
  Register2/1 -> Logical/2
  Logical/1 -> Counter1/1
  const1/1 -> Register1/1, Register2/1
  Register1/1 -> Logical/1
  edge2/1 -> Register2/2
  edge1/1 -> Register1/2

== system PSB_FPGAdesign8_model/Baseband_odd_2/delayCounter_odd_2 ==
  note: Counter that is enabled after the first rising edge1, and disabled after the first rising edge2. Need to calibrate the initial value of counter before getting desired delay value.
  edge1 : Inport
  edge2 : Inport  Port=2
  Counter1 : xbsIndex_r4/Counter  cnt_type=Free Running  cnt_to=Inf  operation=Up  start_count=0  cnt_by_val=1  arith_type=Unsigned  n_bits=12  bin_pt=0  load_pin=off  rst=off  en=on  explicit_period=on  period=1  use_behavioral_HDL=off  implementation=DSP48  dbl_ovrd=off  block_type=counter
  Logical : xbsIndex_r4/Logical  logical_function=XOR  inputs=2  en=off  latency=1  precision=User Defined  arith_type=Boolean  n_bits=1  bin_pt=0  align_bp=on  dbl_ovrd=off  block_type=logical
  Register1 : xbsIndex_r4/Register  init=0  rst=off  en=on  dbl_ovrd=off  block_type=register
  Register2 : xbsIndex_r4/Register  init=0  rst=off  en=on  dbl_ovrd=off  block_type=register
  const1 : xbsIndex_r4/Constant  const=1  gui_display_data_type=Boolean  arith_type=Boolean  n_bits=18  bin_pt=16  preci_type=Single  exp_width=8  frac_width=24  explicit_period=on  period=1  equ=P=C  opselect=C  inp2=PCIN>>17  opr=+  inp1=P  carry=CIN  dbl_ovrd=off  block_type=constant
  delay : Outport
  wires:
  edge1/1 -> Register1/2
  edge2/1 -> Register2/2
  Register1/1 -> Logical/1
  const1/1 -> Register2/1, Register1/1
  Logical/1 -> Counter1/1
  Register2/1 -> Logical/2
  Counter1/1 -> delay/1

== system PSB_FPGAdesign8_model/Baseband_odd_3/delayCounter1 ==
  note: Counter that is enabled after the first rising edge1, and disabled after the first rising edge2. Need to calibrate the initial value of counter before getting desired delay value.
  edge1 : Inport
  edge2 : Inport  Port=2
  Counter1 : xbsIndex_r4/Counter  cnt_type=Free Running  cnt_to=Inf  operation=Up  start_count=0  cnt_by_val=1  arith_type=Unsigned  n_bits=12  bin_pt=0  load_pin=off  rst=off  en=on  explicit_period=on  period=1  use_behavioral_HDL=off  implementation=DSP48  dbl_ovrd=off  block_type=counter
  Logical : xbsIndex_r4/Logical  logical_function=XOR  inputs=2  en=off  latency=1  precision=User Defined  arith_type=Boolean  n_bits=1  bin_pt=0  align_bp=on  dbl_ovrd=off  block_type=logical
  Register1 : xbsIndex_r4/Register  init=0  rst=off  en=on  dbl_ovrd=off  block_type=register
  Register2 : xbsIndex_r4/Register  init=0  rst=off  en=on  dbl_ovrd=off  block_type=register
  const1 : xbsIndex_r4/Constant  const=1  gui_display_data_type=Boolean  arith_type=Boolean  n_bits=18  bin_pt=16  preci_type=Single  exp_width=8  frac_width=24  explicit_period=on  period=1  equ=P=C  opselect=C  inp2=PCIN>>17  opr=+  inp1=P  carry=CIN  dbl_ovrd=off  block_type=constant
  delay : Outport
  wires:
  edge1/1 -> Register1/2
  edge2/1 -> Register2/2
  Register1/1 -> Logical/1
  const1/1 -> Register2/1, Register1/1
  Logical/1 -> Counter1/1
  Register2/1 -> Logical/2
  Counter1/1 -> delay/1

== system PSB_FPGAdesign8_model/Baseband_odd_4/delayCounter_odd_2 ==
  note: Counter that is enabled after the first rising edge1, and disabled after the first rising edge2. Need to calibrate the initial value of counter before getting desired delay value.
  edge1 : Inport
  edge2 : Inport  Port=2
  Counter1 : xbsIndex_r4/Counter  cnt_type=Free Running  cnt_to=Inf  operation=Up  start_count=0  cnt_by_val=1  arith_type=Unsigned  n_bits=12  bin_pt=0  load_pin=off  rst=off  en=on  explicit_period=on  period=1  use_behavioral_HDL=off  implementation=DSP48  dbl_ovrd=off  block_type=counter
  Logical : xbsIndex_r4/Logical  logical_function=XOR  inputs=2  en=off  latency=1  precision=User Defined  arith_type=Boolean  n_bits=1  bin_pt=0  align_bp=on  dbl_ovrd=off  block_type=logical
  Register1 : xbsIndex_r4/Register  init=0  rst=off  en=on  dbl_ovrd=off  block_type=register
  Register2 : xbsIndex_r4/Register  init=0  rst=off  en=on  dbl_ovrd=off  block_type=register
  const1 : xbsIndex_r4/Constant  const=1  gui_display_data_type=Boolean  arith_type=Boolean  n_bits=18  bin_pt=16  preci_type=Single  exp_width=8  frac_width=24  explicit_period=on  period=1  equ=P=C  opselect=C  inp2=PCIN>>17  opr=+  inp1=P  carry=CIN  dbl_ovrd=off  block_type=constant
  delay : Outport
  wires:
  Counter1/1 -> delay/1
  Register2/1 -> Logical/2
  Logical/1 -> Counter1/1
  const1/1 -> Register1/1, Register2/1
  Register1/1 -> Logical/1
  edge2/1 -> Register2/2
  edge1/1 -> Register1/2

== system PSB_FPGAdesign8_model/ToneSelect/FIFO_delay ==
  In1 : Inport
  Constant17 : xbsIndex_r4/Constant  const=1  gui_display_data_type=Boolean  arith_type=Boolean  n_bits=16  bin_pt=14  preci_type=Single  exp_width=8  frac_width=24  explicit_period=on  period=1  equ=P=C  opselect=C  inp2=PCIN>>17  opr=+  inp1=P  carry=CIN  dbl_ovrd=off  block_type=constant
  Delay49 : xbsIndex_r4/Delay  rst=off  infoeditControl=Selection of Reset will increase slice count due to use of real FFs and instead of SRLs  en=off  latency=(6+256)-1  reg_retiming=off  dbl_ovrd=off  block_type=delay
  FIFO3 : xbsIndex_r4/FIFO  mem_type=Block RAM  performance_options=Standard_FIFO  embedded_registers=off  depth=1K  percent_nbits=1  rst=off  rst_latency=2  en=off  use_dcount=off  use_percent_full_port=off  use_almost_empty=off  almost_empty_thresh=2  use_almost_full=off  use_rd_rst_busy=off  use_wr_rst_busy=off  almost_full_thresh=14  explicit_period=off  dbl_ovrd=off  simulation_type=fast_sim  block_type=fifo
  Terminator13 : Terminator
  Terminator14 : Terminator
  Out1 : Outport
  wires:
  FIFO3/2 -> Terminator13/1
  In1/1 -> FIFO3/1
  Constant17/1 -> Delay49/1, FIFO3/2
  Delay49/1 -> FIFO3/3
  FIFO3/3 -> Terminator14/1
  FIFO3/1 -> Out1/1

== system PSB_FPGAdesign8_model/ToneSelect/FIFO_delay1 ==
  In1 : Inport
  Constant17 : xbsIndex_r4/Constant  const=1  gui_display_data_type=Boolean  arith_type=Boolean  n_bits=16  bin_pt=14  preci_type=Single  exp_width=8  frac_width=24  explicit_period=on  period=1  equ=P=C  opselect=C  inp2=PCIN>>17  opr=+  inp1=P  carry=CIN  dbl_ovrd=off  block_type=constant
  Delay49 : xbsIndex_r4/Delay  rst=off  infoeditControl=Selection of Reset will increase slice count due to use of real FFs and instead of SRLs  en=off  latency=(6+256)-1  reg_retiming=off  dbl_ovrd=off  block_type=delay
  FIFO3 : xbsIndex_r4/FIFO  mem_type=Block RAM  performance_options=Standard_FIFO  embedded_registers=off  depth=1K  percent_nbits=1  rst=off  rst_latency=2  en=off  use_dcount=off  use_percent_full_port=off  use_almost_empty=off  almost_empty_thresh=2  use_almost_full=off  use_rd_rst_busy=off  use_wr_rst_busy=off  almost_full_thresh=14  explicit_period=off  dbl_ovrd=off  simulation_type=fast_sim  block_type=fifo
  Terminator13 : Terminator
  Terminator14 : Terminator
  Out1 : Outport
  wires:
  FIFO3/2 -> Terminator13/1
  In1/1 -> FIFO3/1
  Constant17/1 -> Delay49/1, FIFO3/2
  Delay49/1 -> FIFO3/3
  FIFO3/3 -> Terminator14/1
  FIFO3/1 -> Out1/1

== system PSB_FPGAdesign8_model/ToneSelect/FIFO_delay10 ==
  In1 : Inport
  Constant17 : xbsIndex_r4/Constant  const=1  gui_display_data_type=Boolean  arith_type=Boolean  n_bits=16  bin_pt=14  preci_type=Single  exp_width=8  frac_width=24  explicit_period=on  period=1  equ=P=C  opselect=C  inp2=PCIN>>17  opr=+  inp1=P  carry=CIN  dbl_ovrd=off  block_type=constant
  Delay49 : xbsIndex_r4/Delay  rst=off  infoeditControl=Selection of Reset will increase slice count due to use of real FFs and instead of SRLs  en=off  latency=(6+256)-1  reg_retiming=off  dbl_ovrd=off  block_type=delay
  FIFO3 : xbsIndex_r4/FIFO  mem_type=Block RAM  performance_options=Standard_FIFO  embedded_registers=off  depth=1K  percent_nbits=1  rst=off  rst_latency=2  en=off  use_dcount=off  use_percent_full_port=off  use_almost_empty=off  almost_empty_thresh=2  use_almost_full=off  use_rd_rst_busy=off  use_wr_rst_busy=off  almost_full_thresh=14  explicit_period=off  dbl_ovrd=off  simulation_type=fast_sim  block_type=fifo
  Terminator13 : Terminator
  Terminator14 : Terminator
  Out1 : Outport
  wires:
  FIFO3/2 -> Terminator13/1
  In1/1 -> FIFO3/1
  Constant17/1 -> Delay49/1, FIFO3/2
  Delay49/1 -> FIFO3/3
  FIFO3/3 -> Terminator14/1
  FIFO3/1 -> Out1/1

== system PSB_FPGAdesign8_model/ToneSelect/FIFO_delay11 ==
  In1 : Inport
  Constant17 : xbsIndex_r4/Constant  const=1  gui_display_data_type=Boolean  arith_type=Boolean  n_bits=16  bin_pt=14  preci_type=Single  exp_width=8  frac_width=24  explicit_period=on  period=1  equ=P=C  opselect=C  inp2=PCIN>>17  opr=+  inp1=P  carry=CIN  dbl_ovrd=off  block_type=constant
  Delay49 : xbsIndex_r4/Delay  rst=off  infoeditControl=Selection of Reset will increase slice count due to use of real FFs and instead of SRLs  en=off  latency=(6+256)-1  reg_retiming=off  dbl_ovrd=off  block_type=delay
  FIFO3 : xbsIndex_r4/FIFO  mem_type=Block RAM  performance_options=Standard_FIFO  embedded_registers=off  depth=1K  percent_nbits=1  rst=off  rst_latency=2  en=off  use_dcount=off  use_percent_full_port=off  use_almost_empty=off  almost_empty_thresh=2  use_almost_full=off  use_rd_rst_busy=off  use_wr_rst_busy=off  almost_full_thresh=14  explicit_period=off  dbl_ovrd=off  simulation_type=fast_sim  block_type=fifo
  Terminator13 : Terminator
  Terminator14 : Terminator
  Out1 : Outport
  wires:
  FIFO3/2 -> Terminator13/1
  In1/1 -> FIFO3/1
  Constant17/1 -> Delay49/1, FIFO3/2
  Delay49/1 -> FIFO3/3
  FIFO3/3 -> Terminator14/1
  FIFO3/1 -> Out1/1

== system PSB_FPGAdesign8_model/ToneSelect/FIFO_delay12 ==
  In1 : Inport
  Constant17 : xbsIndex_r4/Constant  const=1  gui_display_data_type=Boolean  arith_type=Boolean  n_bits=16  bin_pt=14  preci_type=Single  exp_width=8  frac_width=24  explicit_period=on  period=1  equ=P=C  opselect=C  inp2=PCIN>>17  opr=+  inp1=P  carry=CIN  dbl_ovrd=off  block_type=constant
  Delay49 : xbsIndex_r4/Delay  rst=off  infoeditControl=Selection of Reset will increase slice count due to use of real FFs and instead of SRLs  en=off  latency=(6+256)-1  reg_retiming=off  dbl_ovrd=off  block_type=delay
  FIFO3 : xbsIndex_r4/FIFO  mem_type=Block RAM  performance_options=Standard_FIFO  embedded_registers=off  depth=1K  percent_nbits=1  rst=off  rst_latency=2  en=off  use_dcount=off  use_percent_full_port=off  use_almost_empty=off  almost_empty_thresh=2  use_almost_full=off  use_rd_rst_busy=off  use_wr_rst_busy=off  almost_full_thresh=14  explicit_period=off  dbl_ovrd=off  simulation_type=fast_sim  block_type=fifo
  Terminator13 : Terminator
  Terminator14 : Terminator
  Out1 : Outport
  wires:
  FIFO3/2 -> Terminator13/1
  In1/1 -> FIFO3/1
  Constant17/1 -> Delay49/1, FIFO3/2
  Delay49/1 -> FIFO3/3
  FIFO3/3 -> Terminator14/1
  FIFO3/1 -> Out1/1

== system PSB_FPGAdesign8_model/ToneSelect/FIFO_delay13 ==
  In1 : Inport
  Constant17 : xbsIndex_r4/Constant  const=1  gui_display_data_type=Boolean  arith_type=Boolean  n_bits=16  bin_pt=14  preci_type=Single  exp_width=8  frac_width=24  explicit_period=on  period=1  equ=P=C  opselect=C  inp2=PCIN>>17  opr=+  inp1=P  carry=CIN  dbl_ovrd=off  block_type=constant
  Delay49 : xbsIndex_r4/Delay  rst=off  infoeditControl=Selection of Reset will increase slice count due to use of real FFs and instead of SRLs  en=off  latency=(6+256)-1  reg_retiming=off  dbl_ovrd=off  block_type=delay
  FIFO3 : xbsIndex_r4/FIFO  mem_type=Block RAM  performance_options=Standard_FIFO  embedded_registers=off  depth=1K  percent_nbits=1  rst=off  rst_latency=2  en=off  use_dcount=off  use_percent_full_port=off  use_almost_empty=off  almost_empty_thresh=2  use_almost_full=off  use_rd_rst_busy=off  use_wr_rst_busy=off  almost_full_thresh=14  explicit_period=off  dbl_ovrd=off  simulation_type=fast_sim  block_type=fifo
  Terminator13 : Terminator
  Terminator14 : Terminator
  Out1 : Outport
  wires:
  FIFO3/2 -> Terminator13/1
  In1/1 -> FIFO3/1
  Constant17/1 -> Delay49/1, FIFO3/2
  Delay49/1 -> FIFO3/3
  FIFO3/3 -> Terminator14/1
  FIFO3/1 -> Out1/1

== system PSB_FPGAdesign8_model/ToneSelect/FIFO_delay14 ==
  In1 : Inport
  Constant17 : xbsIndex_r4/Constant  const=1  gui_display_data_type=Boolean  arith_type=Boolean  n_bits=16  bin_pt=14  preci_type=Single  exp_width=8  frac_width=24  explicit_period=on  period=1  equ=P=C  opselect=C  inp2=PCIN>>17  opr=+  inp1=P  carry=CIN  dbl_ovrd=off  block_type=constant
  Delay49 : xbsIndex_r4/Delay  rst=off  infoeditControl=Selection of Reset will increase slice count due to use of real FFs and instead of SRLs  en=off  latency=(6+256)-1  reg_retiming=off  dbl_ovrd=off  block_type=delay
  FIFO3 : xbsIndex_r4/FIFO  mem_type=Block RAM  performance_options=Standard_FIFO  embedded_registers=off  depth=1K  percent_nbits=1  rst=off  rst_latency=2  en=off  use_dcount=off  use_percent_full_port=off  use_almost_empty=off  almost_empty_thresh=2  use_almost_full=off  use_rd_rst_busy=off  use_wr_rst_busy=off  almost_full_thresh=14  explicit_period=off  dbl_ovrd=off  simulation_type=fast_sim  block_type=fifo
  Terminator13 : Terminator
  Terminator14 : Terminator
  Out1 : Outport
  wires:
  FIFO3/2 -> Terminator13/1
  In1/1 -> FIFO3/1
  Constant17/1 -> Delay49/1, FIFO3/2
  Delay49/1 -> FIFO3/3
  FIFO3/3 -> Terminator14/1
  FIFO3/1 -> Out1/1
